simulink model "ARC_DTm"  (R2025b)
settings: Solver=FixedStepAuto  StartTime=0.0  StopTime=10080  FixedStep=1  RelTol=1e-3
PreLoadFcn:
  | %For Preload, set the working path
  | modelFolder = fileparts(which(bdroot));
  | addpath(genpath(modelFolder));
StartFcn:
  | tic
StopFcn:
  | fprintf("Sim Time: %.02f min", toc/60)
values from neighbouring files (symbols this model uses):
  batteryScenario = p.batteryScenario    [RUNSIM_ParameterSweep.m]    (also in _RUNSIM_ParameterSweep.m)
  Electricity_SalePriceModifier = 50/100    (= 0.5)    [RUNSIM_ParameterSweep.m]    (also in _RUNSIM_ParameterSweep.m)
  LUT = LUT_load.gamLUT    [RUNSIM_ParameterSweep.m]    (also in _RUNSIM_ParameterSweep.m)
  minimum_UF_system_flow = 5833    [RUNSIM_ParameterSweep.m]    (also in _RUNSIM_ParameterSweep.m)
  PROS1_recoveryrate = 61    [RUNSIM_ParameterSweep.m]    (also in _RUNSIM_ParameterSweep.m)
  PROS2_recoveryrate = 62    [RUNSIM_ParameterSweep.m]    (also in _RUNSIM_ParameterSweep.m)
  ROstabilization_time = p.ROstabilization_time    [RUNSIM_ParameterSweep.m]    (also in _RUNSIM_ParameterSweep.m)
  solarModifier = maximum_solar_generation / 300    [RUNSIM_ParameterSweep.m]    (also in _RUNSIM_ParameterSweep.m)
  TSRO_recoveryrate = 51    [RUNSIM_ParameterSweep.m]    (also in _RUNSIM_ParameterSweep.m)
  UF_RecoveryRate = 96    [RUNSIM_ParameterSweep.m]    (also in _RUNSIM_ParameterSweep.m)
undefined symbols (not defined in the file or in its folder): A_PROS1, A_PROS2, A_TSRO, B_PROS1, B_PROS2, B_TSRO, BW_Max_Time, BW_Max_Vol_gal, CEB_Max_Time, CEB_Max_Vol_gal, CIP_Max_Time, E, FF, h, L, w
libraries: simulink x40
(part 2 of 11)

== system ARC_DTm/PROS2_1 ==
  note: Units needed:
      | u = cm/sec
      | dh = cm
      | Concentrations = g/L
      | Jw_prev = L/m2/min
      |  = Q (Lpm) / Atot(m2)
      | T = oC
      | q = cm/sec =
      | Q (m3/sec) / Atot (m2)
  Inflow : Inport
  Brine Flow (gpm) : Sum  Inputs=-+
  Bus Creator : BusCreator  Inputs=2
  Bus Creator1 : BusCreator  Inputs=3
  Bus Selector : BusSelector  OutputSignals=S2 Feed Pressure (bar),Feed Temperature (oC),PROS1_1_BrineConductivity_gL,PROS1_1_BrineFlow_gpm
  Bus Selector1 : BusSelector  OutputSignals=PROS2_A,PROS2_B,PROS2_Area_m2
  Channel Area (m2) : Product  Inputs=4
  Check Valve1 : Saturate  UpperLimit=Inf  LowerLimit=0
  Check Valve2 : Saturate  UpperLimit=Inf  LowerLimit=0
  Elements per Vessel : Constant  Value=7
  Feed Channel Height (m) : Constant  Value=L
  Fouling Factor : Constant  Value=1-FF
  Gain : Gain  Gain=3.785
  Initial units : Gain  Gain=10^-8
  Jw_Previous : Memory  InitialCondition=.2949
  "L -> gal" : Gain  Gain=1/3.785
  L>m3 : Gain  Gain=1/1000
  MATLAB Function1 : MATLAB Function  TreatAsAtomicUnit=on
  MATLAB Function2 : MATLAB Function  TreatAsAtomicUnit=on
  Membrane Width (m) : Constant  Value=w
  Min : MinMax  Inputs=2
  Minus : Sum  Inputs=+-|
  Number of Vessels : Constant  Value=40
  Pa > Bar : Gain  Gain=100000
  Permeate Flow (gpm) : Product
  Product : Product  Inputs=*/
  Product2 : Product
  Q (L/min) : Gain  Gain=3.785
  Scope : Scope
      settings: ActiveDisplayYMinimum=-1  ActiveDisplayYMaximum=1  DataLoggingVariableName=ScopeData76
  Scope5 : Scope  NumInputPorts=3
      settings: ActiveDisplayYMinimum=-21.471979594450474  ActiveDisplayYMaximum=418.08306953365  DataLoggingVariableName=ScopeData74
  Spacer Thickness (mm) : Constant  Value=h
  Subsystem : Subsystem
  bar>psi : Gain  Gain=1/.069
  cperm_previous : Memory  InitialCondition=.008
  gpm > L : Gain  Gain=3.785
  initial Units : Gain  Gain=10^-11
  m/min > cm/sec : Gain  Gain=100/60
  m3 > L : Gain  Gain=1000
  m3 > L1 : Gain  Gain=1000
  m>cm : Gain  Gain=100
  m>mm : Gain  Gain=1000
  mm>  cm : Gain  Gain=.1
  mm>m : Gain  Gain=.001
  psi to Bar : Gain  Gain=.069
  s > min : Gain  Gain=60
  s > min1 : Gain  Gain=60
  PROS2_Permeate : Outport
  PROS2_Brine : Outport  Port=2
  tag scope: PROS2_1_deltaPi=global
  wires:
  m/min > cm/sec/1 -> Subsystem/11(u)
  [PROS2_MembraneConstants] -> Bus Selector1/1
  m3 > L1/1 -> s > min1/1
  Bus Selector/1 -> bar>psi/1, Subsystem/2(<S2 Feed Pressure (bar)>), Scope/1, Min/1  "<S2 Feed Pressure (bar)>"
  Bus Selector1/3 -> Permeate Flow (gpm)/2  "<PROS2_Area_m2>"
  Membrane Width (m)/1 -> Channel Area (m2)/1, m>mm/1
  [RO_PermeatePressure] -> psi to Bar/1  "Permeate Pressure (psi)"
  Inflow/1 -> Bus Selector/1
  Bus Selector1/1 -> initial Units/1  "<PROS2_A>"
  Bus Selector1/2 -> Initial units/1  "<PROS2_B>"
  Permeate Flow (gpm)/1 -> Check Valve2/1  "PROS2_1_PermeateFlow_gpm"
  Bus Selector/2 -> Subsystem/1(<Feed Temperature (oC)>)  "<Feed Temperature (oC)>"
  Bus Selector/3 -> MATLAB Function2/5(cfeed), Subsystem/6(<S2 Feed Salinity (g/L)>)  "<PROS1_1_BrineConductivity_gL>"
  Bus Selector/4 -> Q (L/min)/1, Brine Flow (gpm)/2  "<PROS1_1_BrineFlow_gpm>"
  Product/1 -> m/min > cm/sec/1
  psi to Bar/1 -> Min/2  "Pressure (bar)"
  MATLAB Function2/1(cbrine) -> Bus Creator1/2, Scope5/2  "PROS2_1_BrineConductivity_gL"
  initial Units/1 -> m3 > L/1
  Initial units/1 -> m3 > L1/1
  Spacer Thickness (mm)/1 -> MATLAB Function1/2(h), mm>m/1
  m3 > L/1 -> s > min/1
  Min/1 -> Subsystem/3(Pperm)
  mm>m/1 -> Channel Area (m2)/2
  Channel Area (m2)/1 -> Product/2
  Q (L/min)/1 -> MATLAB Function2/4(Qfeed), L>m3/1  "Qtot (L/min)"
  Bus Creator/1 -> PROS2_Permeate/1  "PRO1_PermeateFlow"
  Number of Vessels/1 -> Channel Area (m2)/3
  s > min/1 -> Pa > Bar/1
  Elements per Vessel/1 -> Channel Area (m2)/4
  s > min1/1 -> Subsystem/5(Salt Perm (L/m2/min))  "Salt Perm (L/m2/min)"
  Fouling Factor/1 -> Product2/2
  m>mm/1 -> MATLAB Function1/1(W)
  L>m3/1 -> Product/1
  Pa > Bar/1 -> Product2/1  "Water Perm (L/m2/min/Bar)"
  MATLAB Function1/1(dh) -> mm>  cm/1
  Feed Channel Height (m)/1 -> m>cm/1
  Jw_Previous/1 -> Subsystem/8(Jw)  "Jw"
  cperm_previous/1 -> Subsystem/7(cperm)  "cperm"
  m>cm/1 -> Subsystem/10(L)
  Product2/1 -> Subsystem/4(Water Perm (L/m2/min/Bar))  "Water Perm (L/m2/min/Bar)"
  Gain/1 -> MATLAB Function2/2(Qperm)  "Predicted Permeate Flow (L/min)"
  mm>  cm/1 -> Subsystem/9(dh)
  Bus Creator1/1 -> PROS2_Brine/1  "PROS2_Feedwater"
  bar>psi/1 -> Minus/1  "PROS2_1_ConcentratePressure_psi"
  Subsystem/1(Permeate Flux Rate (L/min/m2)) -> Jw_Previous/1, "L -> gal"/1  "Permeate Flux Rate* (L/min.m2)"
  Subsystem/2(Permeate Salinity g/L) -> Bus Creator/2, MATLAB Function2/1(cperm), cperm_previous/1  "PROS2_1_PermeateSalinity_gL"
  "L -> gal"/1 -> Permeate Flow (gpm)/1
  Subsystem/3(deltaPi_bar) -> [PROS2_1_deltaPi]
  Brine Flow (gpm)/1 -> Check Valve1/1  "PROS2_1_BrineFlow_gpm"
  gpm > L/1 -> MATLAB Function2/3(Qbrine)
  [PROS2_Suction_PressureDrop_psi] -> Minus/2
  Minus/1 -> Scope5/3, Bus Creator1/3  "PROS2_1_ConcentratePressure_psi"
  Check Valve1/1 -> Bus Creator1/1, Scope5/1, gpm > L/1  "PROS2_1_BrineFlow_gpm"
  Check Valve2/1 -> Bus Creator/1, Gain/1, Brine Flow (gpm)/1  "PROS2_1_PermeateFlow_gpm"

== system ARC_DTm/PROS2_1_Pump ==
  note: Determine Needed Added Pressure
  note: gpm / (gpm/psi*ft2) / ft2
  S2 Feed Flow Rate (gpm) : Inport
  Bar > psi : Gain  Gain=1/.069
  Bus Creator : BusCreator  Inputs=4
  Bus Selector : BusSelector  OutputSignals=PROS2_A,PROS2_Area_m2
  Bus Selector1 : BusSelector  OutputSignals=PROS1_1_BrineFlow_gpm,PROS1_1_BrineConductivity_gL,PROS1_1_ConcentratePressure_psi
  Constant2 : Constant  Value=0
  Constant4 : Constant  Value=0
  Gain : Gain  Gain=.01
  Gain3 : Gain  Gain=10.76
  MATLAB Function1 : MATLAB Function  TreatAsAtomicUnit=on
  Max : MinMax  Function=max  Inputs=2
  Memory : Memory  InitialCondition=15
  PROS2_1_recoveryrate_per : Constant  Value=62
  Pa > psi : Gain  Gain=6895
  Product : Product  Inputs=**/
  Product1 : Product
  Sum : Sum  Inputs=|-+
  Sum1 : Sum  Inputs=|++
  Sum2 : Sum  Inputs=|++
  Sum3 : Sum  Inputs=|+-
  Switch : Switch  Criteria=u2 > Threshold  Threshold=1  SaturateOnIntegerOverflow=off  InputSameDT=off
  Switch1 : Switch  Criteria=u2 > Threshold  Threshold=1  SaturateOnIntegerOverflow=off  InputSameDT=off
  m2 > ft2 : Gain  Gain=1/10.76
  m3 > gal : Gain  Gain=264.2
  m3/m2/s/Pa : Gain  Gain=10^-11
  psi to Bar : Gain  Gain=.069
  psi>ft : Gain  Gain=2.31
  s > min : Gain  Gain=60
  PROS2_1_Feedwater : Outport
  tag scope: PROS2_1_Power_kW=global
  wires:
  S2 Feed Flow Rate (gpm)/1 -> Bus Selector1/1  "InflowRate (gpm)"
  Sum1/1 -> Sum2/1  "Net Opposing Pressure (psi)"
  [PROS2_MembraneConstants] -> Bus Selector/1
  Pa > psi/1 -> m2 > ft2/1  "Water Perm (gpm/m2/bar)"
  Sum2/1 -> psi to Bar/1, Sum/2  "PROS2_1_FeedPressure_psi"
  m3 > gal/1 -> s > min/1
  [T] -> Bus Creator/2  "Feed Temperature (oC)"
  Memory/1 -> Sum1/1
  Product/1 -> Sum2/2  "PROS2_1_RequiredNDP_psi"
  PROS2_1_recoveryrate_per/1 -> Gain/1
  psi to Bar/1 -> Bus Creator/4  "S2 Feed Pressure (bar)"
  Gain3/1 -> Product1/2  "PROS2_Area_ft2"
  m2 > ft2/1 -> Product1/1  "PROS2_WaterPermeability_gpm_psi_ft2"
  Sum/1 -> psi>ft/1
  m3/m2/s/Pa/1 -> m3 > gal/1
  Bus Selector/1 -> m3/m2/s/Pa/1  "<PROS2_A>"
  Product1/1 -> Product/3
  [PROS2_1_deltaPi] -> Bar > psi/1
  Gain/1 -> Product/2
  s > min/1 -> Pa > psi/1
  Bar > psi/1 -> Memory/1
  Bus Creator/1 -> PROS2_1_Feedwater/1
  psi>ft/1 -> MATLAB Function1/2(h_des)
  Bus Selector1/2 -> Bus Creator/1  "<PROS1_1_BrineConductivity_gL>"
  Max/1 -> Sum3/1
  Bus Selector/2 -> Gain3/1  "<PROS2_Area_m2>"
  Sum3/1 -> Sum/1
  [PROS2_Suction_PressureDrop_psi] -> Switch1/1
  MATLAB Function1/2(power) -> [PROS2_1_Power_kW]  "PROS2_1_Power_kW"
  Bus Selector1/3 -> Max/1  "<PROS1_1_ConcentratePressure_psi>"
  Constant2/1 -> Switch1/3, Max/2
  Bus Selector1/1 -> Switch1/2, MATLAB Function1/1(Q_des), Bus Creator/3, Switch/2, Product/1  "<PROS1_1_BrineFlow_gpm>"
  [RO_PermeatePressure] -> Switch/1
  Constant4/1 -> Switch/3
  Switch/1 -> Sum1/2
  Switch1/1 -> Sum3/2

== system ARC_DTm/PROS2_2 ==
  note: Units needed:
      | u = cm/sec
      | dh = cm
      | Concentrations = g/L
      | Jw_prev = L/m2/min
      |  = Q (Lpm) / Atot(m2)
      | T = oC
      | q = cm/sec =
      | Q (m3/sec) / Atot (m2)
  Inflow : Inport
  Brine Flow (gpm) : Sum  Inputs=-+
  Bus Creator : BusCreator  Inputs=2
  Bus Creator1 : BusCreator  Inputs=3
  Bus Selector : BusSelector  OutputSignals=S2 Feed Pressure (bar),Feed Temperature (oC),PROS1_2_BrineConductivity_gL,PROS1_2_BrineFlow_gpm
  Bus Selector1 : BusSelector  OutputSignals=PROS2_A,PROS2_B,PROS2_Area_m2
  Channel Area (m2) : Product  Inputs=4
  Check Valve : Saturate  UpperLimit=Inf  LowerLimit=0
  Check Valve1 : Saturate  UpperLimit=Inf  LowerLimit=0
  Elements per Vessel : Constant  Value=7
  Feed Channel Height (m) : Constant  Value=L
  Fouling Factor : Constant  Value=1-FF
  Gain : Gain  Gain=3.785
  Initial units : Gain  Gain=10^-8
  Jw_Previous : Memory  InitialCondition=.2949
  "L -> gal" : Gain  Gain=1/3.785
  L>m3 : Gain  Gain=1/1000
  MATLAB Function1 : MATLAB Function  TreatAsAtomicUnit=on
  MATLAB Function2 : MATLAB Function  TreatAsAtomicUnit=on
  Membrane Width (m) : Constant  Value=w
  Min : MinMax  Inputs=2
  Minus : Sum  Inputs=+-|
  Number of Vessels : Constant  Value=40
  Pa > Bar : Gain  Gain=100000
  Permeate Flow (gpm) : Product
  Product : Product  Inputs=*/
  Product2 : Product
  Q (L/min) : Gain  Gain=3.785
  Scope : Scope
      settings: ActiveDisplayYMinimum=-1  ActiveDisplayYMaximum=1  DataLoggingVariableName=ScopeData76
  Scope5 : Scope  NumInputPorts=3
      settings: ActiveDisplayYMinimum=-102.45583996757739  ActiveDisplayYMaximum=443.57810434622803  DataLoggingVariableName=ScopeData74
  Spacer Thickness (mm) : Constant  Value=h
  Subsystem : Subsystem
  bar>psi : Gain  Gain=1/.069
  cperm_previous : Memory  InitialCondition=.008
  gpm > L : Gain  Gain=3.785
  initial Units : Gain  Gain=10^-11
  m/min > cm/sec : Gain  Gain=100/60
  m3 > L : Gain  Gain=1000
  m3 > L1 : Gain  Gain=1000
  m>cm : Gain  Gain=100
  m>mm : Gain  Gain=1000
  mm>  cm : Gain  Gain=.1
  mm>m : Gain  Gain=.001
  psi to Bar : Gain  Gain=.069
  s > min : Gain  Gain=60
  s > min1 : Gain  Gain=60
  PROS2_Permeate : Outport
  PROS2_Brine : Outport  Port=2
  tag scope: PROS2_2_deltaPi=global
  wires:
  m/min > cm/sec/1 -> Subsystem/11(u)
  [PROS2_MembraneConstants] -> Bus Selector1/1
  m3 > L1/1 -> s > min1/1
  Bus Selector/1 -> bar>psi/1, Subsystem/2(<S2 Feed Pressure (bar)>), Scope/1, Min/1  "<S2 Feed Pressure (bar)>"
  Bus Selector1/3 -> Permeate Flow (gpm)/2  "<PROS2_Area_m2>"
  Membrane Width (m)/1 -> Channel Area (m2)/1, m>mm/1
  [RO_PermeatePressure] -> psi to Bar/1  "Permeate Pressure (psi)"
  Inflow/1 -> Bus Selector/1
  Bus Selector1/1 -> initial Units/1  "<PROS2_A>"
  Bus Selector1/2 -> Initial units/1  "<PROS2_B>"
  Permeate Flow (gpm)/1 -> Check Valve/1  "PROS2_2_PermeateFlow_gpm"
  Bus Selector/2 -> Subsystem/1(<Feed Temperature (oC)>)  "<Feed Temperature (oC)>"
  Bus Selector/3 -> MATLAB Function2/5(cfeed), Subsystem/6(<S2 Feed Salinity (g/L)>)  "<PROS1_2_BrineConductivity_gL>"
  Bus Selector/4 -> Q (L/min)/1, Brine Flow (gpm)/2  "<PROS1_2_BrineFlow_gpm>"
  Product/1 -> m/min > cm/sec/1
  psi to Bar/1 -> Min/2  "Pressure (bar)"
  MATLAB Function2/1(cbrine) -> Bus Creator1/2, Scope5/2  "PROS2_2_BrineConductivity_gL"
  initial Units/1 -> m3 > L/1
  Initial units/1 -> m3 > L1/1
  Spacer Thickness (mm)/1 -> MATLAB Function1/2(h), mm>m/1
  m3 > L/1 -> s > min/1
  Min/1 -> Subsystem/3(Pperm)
  mm>m/1 -> Channel Area (m2)/2
  Channel Area (m2)/1 -> Product/2
  Q (L/min)/1 -> MATLAB Function2/4(Qfeed), L>m3/1  "Qtot (L/min)"
  Bus Creator/1 -> PROS2_Permeate/1  "PRO1_PermeateFlow"
  Number of Vessels/1 -> Channel Area (m2)/3
  s > min/1 -> Pa > Bar/1
  Elements per Vessel/1 -> Channel Area (m2)/4
  s > min1/1 -> Subsystem/5(Salt Perm (L/m2/min))  "Salt Perm (L/m2/min)"
  Fouling Factor/1 -> Product2/2
  m>mm/1 -> MATLAB Function1/1(W)
  L>m3/1 -> Product/1
  Pa > Bar/1 -> Product2/1  "Water Perm (L/m2/min/Bar)"
  MATLAB Function1/1(dh) -> mm>  cm/1
  Feed Channel Height (m)/1 -> m>cm/1
  Jw_Previous/1 -> Subsystem/8(Jw)  "Jw"
  cperm_previous/1 -> Subsystem/7(cperm)  "cperm"
  m>cm/1 -> Subsystem/10(L)
  Product2/1 -> Subsystem/4(Water Perm (L/m2/min/Bar))  "Water Perm (L/m2/min/Bar)"
  Gain/1 -> MATLAB Function2/2(Qperm)  "Predicted Permeate Flow (L/min)"
  mm>  cm/1 -> Subsystem/9(dh)
  Bus Creator1/1 -> PROS2_Brine/1  "PROS2_Feedwater"
  bar>psi/1 -> Minus/1  "PROS2_2_ConcentratePressure_psi"
  Subsystem/1(Permeate Flux Rate (L/min/m2)) -> Jw_Previous/1, "L -> gal"/1  "Permeate Flux Rate* (L/min.m2)"
  Subsystem/2(Permeate Salinity g/L) -> Bus Creator/2, MATLAB Function2/1(cperm), cperm_previous/1  "PROS2_2_PermeateSalinity_gL"
  "L -> gal"/1 -> Permeate Flow (gpm)/1
  Subsystem/3(deltaPi_bar) -> [PROS2_2_deltaPi]
  Brine Flow (gpm)/1 -> Check Valve1/1  "PROS2_2_BrineFlow_gpm"
  gpm > L/1 -> MATLAB Function2/3(Qbrine)
  [PROS2_Suction_PressureDrop_psi] -> Minus/2
  Minus/1 -> Scope5/3, Bus Creator1/3  "PROS2_2_ConcentratePressure_psi"
  Check Valve/1 -> Bus Creator/1, Gain/1, Brine Flow (gpm)/1  "PROS2_2_PermeateFlow_gpm"
  Check Valve1/1 -> Bus Creator1/1, Scope5/1, gpm > L/1  "PROS2_2_BrineFlow_gpm"

== system ARC_DTm/PROS2_2_Pump ==
  note: Determine Needed Added Pressure
  note: gpm / (gpm/psi*ft2) / ft2
  S2 Feed Flow Rate (gpm) : Inport
  Bar > psi : Gain  Gain=1/.069
  Bus Creator : BusCreator  Inputs=4
  Bus Selector : BusSelector  OutputSignals=PROS2_A,PROS2_Area_m2
  Bus Selector1 : BusSelector  OutputSignals=PROS1_2_BrineFlow_gpm,PROS1_2_BrineConductivity_gL,PROS1_2_ConcentratePressure_psi
  Constant2 : Constant  Value=0
  Constant4 : Constant  Value=0
  Gain : Gain  Gain=.01
  Gain3 : Gain  Gain=10.76
  MATLAB Function1 : MATLAB Function  TreatAsAtomicUnit=on
  Max : MinMax  Function=max  Inputs=2
  Memory : Memory  InitialCondition=15
  PROS2_2_recoveryrate_per : Constant  Value=62
  Pa > psi : Gain  Gain=6895
  Product : Product  Inputs=**/
  Product1 : Product
  Sum : Sum  Inputs=|-+
  Sum1 : Sum  Inputs=|++
  Sum2 : Sum  Inputs=|++
  Sum3 : Sum  Inputs=|+-
  Switch : Switch  Criteria=u2 > Threshold  Threshold=1  SaturateOnIntegerOverflow=off  InputSameDT=off
  Switch1 : Switch  Criteria=u2 > Threshold  Threshold=1  SaturateOnIntegerOverflow=off  InputSameDT=off
  m2 > ft2 : Gain  Gain=1/10.76
  m3 > gal : Gain  Gain=264.2
  m3/m2/s/Pa : Gain  Gain=10^-11
  psi to Bar : Gain  Gain=.069
  psi>ft : Gain  Gain=2.31
  s > min : Gain  Gain=60
  PROS2_2_Feedwater : Outport
  tag scope: PROS2_2_Power_kW=global
  wires:
  S2 Feed Flow Rate (gpm)/1 -> Bus Selector1/1  "InflowRate (gpm)"
  Sum1/1 -> Sum2/1  "Net Opposing Pressure (psi)"
  [PROS2_MembraneConstants] -> Bus Selector/1
  Pa > psi/1 -> m2 > ft2/1  "Water Perm (gpm/m2/bar)"
  Sum2/1 -> psi to Bar/1, Sum/2  "PROS2_2_FeedPressure_psi"
  m3 > gal/1 -> s > min/1
  [T] -> Bus Creator/2  "Feed Temperature (oC)"
  Memory/1 -> Sum1/1
  Product/1 -> Sum2/2  "PROS2_2_RequiredNDP_psi"
  PROS2_2_recoveryrate_per/1 -> Gain/1
  psi to Bar/1 -> Bus Creator/4  "S2 Feed Pressure (bar)"
  Gain3/1 -> Product1/2  "PROS2_Area_ft2"
  m2 > ft2/1 -> Product1/1  "PROS2_WaterPermeability_gpm_psi_ft2"
  Sum/1 -> psi>ft/1
  m3/m2/s/Pa/1 -> m3 > gal/1
  Bus Selector/1 -> m3/m2/s/Pa/1  "<PROS2_A>"
  Product1/1 -> Product/3
  [PROS2_2_deltaPi] -> Bar > psi/1
  Gain/1 -> Product/2
  s > min/1 -> Pa > psi/1
  Bar > psi/1 -> Memory/1
  Bus Creator/1 -> PROS2_2_Feedwater/1
  psi>ft/1 -> MATLAB Function1/2(h_des)
  Bus Selector1/2 -> Bus Creator/1  "<PROS1_2_BrineConductivity_gL>"
  Max/1 -> Sum3/1
  Bus Selector/2 -> Gain3/1  "<PROS2_Area_m2>"
  Sum3/1 -> Sum/1
  [PROS2_Suction_PressureDrop_psi] -> Switch1/1
  MATLAB Function1/2(power) -> [PROS2_2_Power_kW]  "PROS2_2_Power_kW"
  Bus Selector1/3 -> Max/1  "<PROS1_2_ConcentratePressure_psi>"
  Constant2/1 -> Switch1/3, Max/2
  Bus Selector1/1 -> Switch1/2, MATLAB Function1/1(Q_des), Bus Creator/3, Switch/2, Product/1  "<PROS1_2_BrineFlow_gpm>"
  [RO_PermeatePressure] -> Switch/1
  Constant4/1 -> Switch/3
  Switch/1 -> Sum1/2
  Switch1/1 -> Sum3/2

== system ARC_DTm/PROS2_3 ==
  note: Units needed:
      | u = cm/sec
      | dh = cm
      | Concentrations = g/L
      | Jw_prev = L/m2/min
      |  = Q (Lpm) / Atot(m2)
      | T = oC
      | q = cm/sec =
      | Q (m3/sec) / Atot (m2)
  Inflow : Inport
  Brine Flow (gpm) : Sum  Inputs=-+
  Bus Creator : BusCreator  Inputs=2
  Bus Creator1 : BusCreator  Inputs=3
  Bus Selector : BusSelector  OutputSignals=S2 Feed Pressure (bar),Feed Temperature (oC),PROS1_3_BrineConductivity_gL,PROS1_3_BrineFlow_gpm
  Bus Selector1 : BusSelector  OutputSignals=PROS2_A,PROS2_B,PROS2_Area_m2
  Channel Area (m2) : Product  Inputs=4
  Check Valve : Saturate  UpperLimit=Inf  LowerLimit=0
  Check Valve1 : Saturate  UpperLimit=Inf  LowerLimit=0
  Elements per Vessel : Constant  Value=7
  Feed Channel Height (m) : Constant  Value=L
  Fouling Factor : Constant  Value=1-FF
  Gain : Gain  Gain=3.785
  Initial units : Gain  Gain=10^-8
  Jw_Previous : Memory  InitialCondition=.2949
  "L -> gal" : Gain  Gain=1/3.785
  L>m3 : Gain  Gain=1/1000
  MATLAB Function1 : MATLAB Function  TreatAsAtomicUnit=on
  MATLAB Function2 : MATLAB Function  TreatAsAtomicUnit=on
  Membrane Width (m) : Constant  Value=w
  Min : MinMax  Inputs=2
  Minus : Sum  Inputs=+-|
  Number of Vessels : Constant  Value=40
  Pa > Bar : Gain  Gain=100000
  Permeate Flow (gpm) : Product
  Product : Product  Inputs=*/
  Product2 : Product
  Q (L/min) : Gain  Gain=3.785
  Scope : Scope
      settings: ActiveDisplayYMinimum=-1  ActiveDisplayYMaximum=1  DataLoggingVariableName=ScopeData76
  Spacer Thickness (mm) : Constant  Value=h
  Subsystem : Subsystem
  bar>psi : Gain  Gain=1/.069
  cperm_previous : Memory  InitialCondition=.008
  gpm > L : Gain  Gain=3.785
  initial Units : Gain  Gain=10^-11
  m/min > cm/sec : Gain  Gain=100/60
  m3 > L : Gain  Gain=1000
  m3 > L1 : Gain  Gain=1000
  m>cm : Gain  Gain=100
  m>mm : Gain  Gain=1000
  mm>  cm : Gain  Gain=.1
  mm>m : Gain  Gain=.001
  psi to Bar : Gain  Gain=.069
  s > min : Gain  Gain=60
  s > min1 : Gain  Gain=60
  PROS2_Permeate : Outport
  PROS2_Brine : Outport  Port=2
  tag scope: PROS2_3_deltaPi=global
  wires:
  m/min > cm/sec/1 -> Subsystem/11(u)
  [PROS2_MembraneConstants] -> Bus Selector1/1
  m3 > L1/1 -> s > min1/1
  Bus Selector/1 -> bar>psi/1, Subsystem/2(<S2 Feed Pressure (bar)>), Scope/1, Min/1  "<S2 Feed Pressure (bar)>"
  Bus Selector1/3 -> Permeate Flow (gpm)/2  "<PROS2_Area_m2>"
  Membrane Width (m)/1 -> Channel Area (m2)/1, m>mm/1
  [RO_PermeatePressure] -> psi to Bar/1  "Permeate Pressure (psi)"
  Inflow/1 -> Bus Selector/1
  Bus Selector1/1 -> initial Units/1  "<PROS2_A>"
  Bus Selector1/2 -> Initial units/1  "<PROS2_B>"
  Permeate Flow (gpm)/1 -> Check Valve1/1  "PROS2_3_PermeateFlow_gpm"
  Bus Selector/2 -> Subsystem/1(<Feed Temperature (oC)>)  "<Feed Temperature (oC)>"
  Bus Selector/3 -> MATLAB Function2/5(cfeed), Subsystem/6(<S2 Feed Salinity (g/L)>)  "<PROS1_3_BrineConductivity_gL>"
  Bus Selector/4 -> Q (L/min)/1, Brine Flow (gpm)/2  "<PROS1_3_BrineFlow_gpm>"
  Product/1 -> m/min > cm/sec/1
  psi to Bar/1 -> Min/2  "Pressure (bar)"
  MATLAB Function2/1(cbrine) -> Bus Creator1/2  "PROS2_3_BrineConductivity_gL"
  initial Units/1 -> m3 > L/1
  Initial units/1 -> m3 > L1/1
  Spacer Thickness (mm)/1 -> MATLAB Function1/2(h), mm>m/1
  m3 > L/1 -> s > min/1
  Min/1 -> Subsystem/3(Pperm)
  mm>m/1 -> Channel Area (m2)/2
  Channel Area (m2)/1 -> Product/2
  Q (L/min)/1 -> MATLAB Function2/4(Qfeed), L>m3/1  "Qtot (L/min)"
  Bus Creator/1 -> PROS2_Permeate/1  "PRO1_PermeateFlow"
  Number of Vessels/1 -> Channel Area (m2)/3
  s > min/1 -> Pa > Bar/1
  Elements per Vessel/1 -> Channel Area (m2)/4
  s > min1/1 -> Subsystem/5(Salt Perm (L/m2/min))  "Salt Perm (L/m2/min)"
  Fouling Factor/1 -> Product2/2
  m>mm/1 -> MATLAB Function1/1(W)
  L>m3/1 -> Product/1
  Pa > Bar/1 -> Product2/1  "Water Perm (L/m2/min/Bar)"
  MATLAB Function1/1(dh) -> mm>  cm/1
  Feed Channel Height (m)/1 -> m>cm/1
  Jw_Previous/1 -> Subsystem/8(Jw)  "Jw"
  cperm_previous/1 -> Subsystem/7(cperm)  "cperm"
  m>cm/1 -> Subsystem/10(L)
  Product2/1 -> Subsystem/4(Water Perm (L/m2/min/Bar))  "Water Perm (L/m2/min/Bar)"
  Gain/1 -> MATLAB Function2/2(Qperm)  "Predicted Permeate Flow (L/min)"
  mm>  cm/1 -> Subsystem/9(dh)
  Bus Creator1/1 -> PROS2_Brine/1  "PROS2_Feedwater"
  bar>psi/1 -> Minus/1  "PROS2_3_ConcentratePressure_psi"
  Subsystem/1(Permeate Flux Rate (L/min/m2)) -> Jw_Previous/1, "L -> gal"/1  "Permeate Flux Rate* (L/min.m2)"
  Subsystem/2(Permeate Salinity g/L) -> Bus Creator/2, MATLAB Function2/1(cperm), cperm_previous/1  "PROS2_3_PermeateSalinity_gL"
  "L -> gal"/1 -> Permeate Flow (gpm)/1
  Subsystem/3(deltaPi_bar) -> [PROS2_3_deltaPi]
  Check Valve/1 -> Bus Creator1/1, gpm > L/1  "PROS2_3_BrineFlow_gpm"
  gpm > L/1 -> MATLAB Function2/3(Qbrine)
  [PROS2_Suction_PressureDrop_psi] -> Minus/2
  Minus/1 -> Bus Creator1/3  "PROS2_3_ConcentratePressure_psi"
  Brine Flow (gpm)/1 -> Check Valve/1  "PROS2_3_BrineFlow_gpm"
  Check Valve1/1 -> Bus Creator/1, Gain/1, Brine Flow (gpm)/1  "PROS2_3_PermeateFlow_gpm"

== system ARC_DTm/PROS2_3_Pump ==
  note: Determine Needed Added Pressure
  note: gpm / (gpm/psi*ft2) / ft2
  S2 Feed Flow Rate (gpm) : Inport
  Bar > psi : Gain  Gain=1/.069
  Bus Creator : BusCreator  Inputs=4
  Bus Selector : BusSelector  OutputSignals=PROS2_A,PROS2_Area_m2
  Bus Selector1 : BusSelector  OutputSignals=PROS1_3_BrineFlow_gpm,PROS1_3_BrineConductivity_gL,PROS1_3_ConcentratePressure_psi
  Constant2 : Constant  Value=0
  Constant4 : Constant  Value=0
  Gain : Gain  Gain=.01
  Gain3 : Gain  Gain=10.76
  MATLAB Function1 : MATLAB Function  TreatAsAtomicUnit=on
  Max : MinMax  Function=max  Inputs=2
  Memory : Memory  InitialCondition=15
  PROS2_3_recoveryrate_per : Constant  Value=62
  Pa > psi : Gain  Gain=6895
  Product : Product  Inputs=**/
  Product1 : Product
  Sum : Sum  Inputs=|-+
  Sum1 : Sum  Inputs=|++
  Sum2 : Sum  Inputs=|++
  Sum3 : Sum  Inputs=|+-
  Switch : Switch  Criteria=u2 > Threshold  Threshold=1  SaturateOnIntegerOverflow=off  InputSameDT=off
  Switch1 : Switch  Criteria=u2 > Threshold  Threshold=1  SaturateOnIntegerOverflow=off  InputSameDT=off
  m2 > ft2 : Gain  Gain=1/10.76
  m3 > gal : Gain  Gain=264.2
  m3/m2/s/Pa : Gain  Gain=10^-11
  psi to Bar : Gain  Gain=.069
  psi>ft : Gain  Gain=2.31
  s > min : Gain  Gain=60
  PROS2_3_Feedwater : Outport
  tag scope: PROS2_3_Power_kW=global
  wires:
  S2 Feed Flow Rate (gpm)/1 -> Bus Selector1/1  "InflowRate (gpm)"
  Sum1/1 -> Sum2/1  "Net Opposing Pressure (psi)"
  [PROS2_MembraneConstants] -> Bus Selector/1
  Pa > psi/1 -> m2 > ft2/1  "Water Perm (gpm/m2/bar)"
  Sum2/1 -> psi to Bar/1, Sum/2  "PROS2_3_FeedPressure_psi"
  m3 > gal/1 -> s > min/1
  [T] -> Bus Creator/2  "Feed Temperature (oC)"
  Memory/1 -> Sum1/1
  Product/1 -> Sum2/2  "PROS2_3_RequiredNDP_psi"
  PROS2_3_recoveryrate_per/1 -> Gain/1
  psi to Bar/1 -> Bus Creator/4  "S2 Feed Pressure (bar)"
  Gain3/1 -> Product1/2  "PROS2_Area_ft2"
  m2 > ft2/1 -> Product1/1  "PROS2_WaterPermeability_gpm_psi_ft2"
  Sum/1 -> psi>ft/1
  m3/m2/s/Pa/1 -> m3 > gal/1
  Bus Selector/1 -> m3/m2/s/Pa/1  "<PROS2_A>"
  Product1/1 -> Product/3
  [PROS2_3_deltaPi] -> Bar > psi/1
  Gain/1 -> Product/2
  s > min/1 -> Pa > psi/1
  Bar > psi/1 -> Memory/1
  Bus Creator/1 -> PROS2_3_Feedwater/1
  psi>ft/1 -> MATLAB Function1/2(h_des)
  Bus Selector1/2 -> Bus Creator/1  "<PROS1_3_BrineConductivity_gL>"
  Max/1 -> Sum3/1
  Bus Selector/2 -> Gain3/1  "<PROS2_Area_m2>"
  Sum3/1 -> Sum/1
  [PROS2_Suction_PressureDrop_psi] -> Switch1/1
  MATLAB Function1/2(power) -> [PROS2_3_Power_kW]  "PROS2_3_Power_kW"
  Bus Selector1/3 -> Max/1  "<PROS1_3_ConcentratePressure_psi>"
  Constant2/1 -> Switch1/3, Max/2
  Bus Selector1/1 -> Switch1/2, MATLAB Function1/1(Q_des), Bus Creator/3, Switch/2, Product/1  "<PROS1_3_BrineFlow_gpm>"
  [RO_PermeatePressure] -> Switch/1
  Constant4/1 -> Switch/3
  Switch/1 -> Sum1/2
  Switch1/1 -> Sum3/2

== system ARC_DTm/PROS2_4 ==
  note: Units needed:
      | u = cm/sec
      | dh = cm
      | Concentrations = g/L
      | Jw_prev = L/m2/min
      |  = Q (Lpm) / Atot(m2)
      | T = oC
      | q = cm/sec =
      | Q (m3/sec) / Atot (m2)
  Inflow : Inport
  Brine Flow (gpm) : Sum  Inputs=-+
  Bus Creator : BusCreator  Inputs=2
  Bus Creator1 : BusCreator  Inputs=3
  Bus Selector : BusSelector  OutputSignals=S2 Feed Pressure (bar),Feed Temperature (oC),PROS1_4_BrineConductivity_gL,PROS1_4_BrineFlow_gpm
  Bus Selector1 : BusSelector  OutputSignals=PROS2_A,PROS2_B,PROS2_Area_m2
  Channel Area (m2) : Product  Inputs=4
  Check Valve : Saturate  UpperLimit=Inf  LowerLimit=0
  Check Valve2 : Saturate  UpperLimit=Inf  LowerLimit=0
  Elements per Vessel : Constant  Value=7
  Feed Channel Height (m) : Constant  Value=L
  Fouling Factor : Constant  Value=1-FF
  Gain : Gain  Gain=3.785
  Initial units : Gain  Gain=10^-8
  Jw_Previous : Memory  InitialCondition=.2949
  "L -> gal" : Gain  Gain=1/3.785
  L>m3 : Gain  Gain=1/1000
  MATLAB Function1 : MATLAB Function  TreatAsAtomicUnit=on
  MATLAB Function2 : MATLAB Function  TreatAsAtomicUnit=on
  Membrane Width (m) : Constant  Value=w
  Min : MinMax  Inputs=2
  Minus : Sum  Inputs=+-|
  Number of Vessels : Constant  Value=40
  Pa > Bar : Gain  Gain=100000
  Permeate Flow (gpm) : Product
  Product : Product  Inputs=*/
  Product2 : Product
  Q (L/min) : Gain  Gain=3.785
  Scope : Scope
      settings: ActiveDisplayYMinimum=-1  ActiveDisplayYMaximum=1  DataLoggingVariableName=ScopeData76
  Scope1 : Scope  NumInputPorts=2
      settings: ActiveDisplayYMinimum=-394.68314201102044  ActiveDisplayYMaximum=456.3600674223589  DataLoggingVariableName=ScopeData35
  Spacer Thickness (mm) : Constant  Value=h
  Subsystem : Subsystem
  bar>psi : Gain  Gain=1/.069
  cperm_previous : Memory  InitialCondition=.008
  gpm > L : Gain  Gain=3.785
  initial Units : Gain  Gain=10^-11
  m/min > cm/sec : Gain  Gain=100/60
  m3 > L : Gain  Gain=1000
  m3 > L1 : Gain  Gain=1000
  m>cm : Gain  Gain=100
  m>mm : Gain  Gain=1000
  mm>  cm : Gain  Gain=.1
  mm>m : Gain  Gain=.001
  psi to Bar : Gain  Gain=.069
  s > min : Gain  Gain=60
  s > min1 : Gain  Gain=60
  PROS2_Permeate : Outport
  PROS2_Brine : Outport  Port=2
  tag scope: PROS2_4_deltaPi=global
  wires:
  m/min > cm/sec/1 -> Subsystem/11(u)
  [PROS2_MembraneConstants] -> Bus Selector1/1
  m3 > L1/1 -> s > min1/1
  Bus Selector/1 -> bar>psi/1, Subsystem/2(<S2 Feed Pressure (bar)>), Scope/1, Min/1  "<S2 Feed Pressure (bar)>"
  Bus Selector1/3 -> Permeate Flow (gpm)/2  "<PROS2_Area_m2>"
  Membrane Width (m)/1 -> Channel Area (m2)/1, m>mm/1
  [RO_PermeatePressure] -> psi to Bar/1  "Permeate Pressure (psi)"
  Inflow/1 -> Bus Selector/1
  Bus Selector1/1 -> initial Units/1  "<PROS2_A>"
  Bus Selector1/2 -> Initial units/1  "<PROS2_B>"
  Permeate Flow (gpm)/1 -> Check Valve2/1  "PROS2_4_PermeateFlow_gpm"
  Bus Selector/2 -> Subsystem/1(<Feed Temperature (oC)>)  "<Feed Temperature (oC)>"
  Bus Selector/3 -> MATLAB Function2/5(cfeed), Subsystem/6(<S2 Feed Salinity (g/L)>)  "<PROS1_4_BrineConductivity_gL>"
  Bus Selector/4 -> Q (L/min)/1, Brine Flow (gpm)/2  "<PROS1_4_BrineFlow_gpm>"
  Product/1 -> m/min > cm/sec/1
  psi to Bar/1 -> Min/2  "Pressure (bar)"
  MATLAB Function2/1(cbrine) -> Scope1/2, Bus Creator1/2  "PROS2_4_BrineConductivity_gL"
  initial Units/1 -> m3 > L/1
  Initial units/1 -> m3 > L1/1
  Spacer Thickness (mm)/1 -> MATLAB Function1/2(h), mm>m/1
  m3 > L/1 -> s > min/1
  Min/1 -> Subsystem/3(Pperm)
  mm>m/1 -> Channel Area (m2)/2
  Channel Area (m2)/1 -> Product/2
  Q (L/min)/1 -> MATLAB Function2/4(Qfeed), L>m3/1  "Qtot (L/min)"
  Bus Creator/1 -> PROS2_Permeate/1  "PRO1_PermeateFlow"
  Number of Vessels/1 -> Channel Area (m2)/3
  s > min/1 -> Pa > Bar/1
  Elements per Vessel/1 -> Channel Area (m2)/4
  s > min1/1 -> Subsystem/5(Salt Perm (L/m2/min))  "Salt Perm (L/m2/min)"
  Fouling Factor/1 -> Product2/2
  m>mm/1 -> MATLAB Function1/1(W)
  L>m3/1 -> Product/1
  Pa > Bar/1 -> Product2/1  "Water Perm (L/m2/min/Bar)"
  MATLAB Function1/1(dh) -> mm>  cm/1
  Feed Channel Height (m)/1 -> m>cm/1
  Jw_Previous/1 -> Subsystem/8(Jw)  "Jw"
  cperm_previous/1 -> Subsystem/7(cperm)  "cperm"
  m>cm/1 -> Subsystem/10(L)
  Product2/1 -> Subsystem/4(Water Perm (L/m2/min/Bar))  "Water Perm (L/m2/min/Bar)"
  Gain/1 -> MATLAB Function2/2(Qperm)  "Predicted Permeate Flow (L/min)"
  mm>  cm/1 -> Subsystem/9(dh)
  Bus Creator1/1 -> PROS2_Brine/1  "PROS2_Feedwater"
  bar>psi/1 -> Minus/1  "PROS2_4_ConcentratePressure_psi"
  Subsystem/1(Permeate Flux Rate (L/min/m2)) -> Jw_Previous/1, "L -> gal"/1  "Permeate Flux Rate* (L/min.m2)"
  Subsystem/2(Permeate Salinity g/L) -> Bus Creator/2, MATLAB Function2/1(cperm), cperm_previous/1  "PROS2_4_PermeateSalinity_gL"
  "L -> gal"/1 -> Permeate Flow (gpm)/1
  Subsystem/3(deltaPi_bar) -> [PROS2_4_deltaPi]
  Check Valve/1 -> Bus Creator1/1, Scope1/1, gpm > L/1  "PROS2_4_BrineFlow_gpm"
  gpm > L/1 -> MATLAB Function2/3(Qbrine)
  [PROS2_Suction_PressureDrop_psi] -> Minus/2
  Minus/1 -> Bus Creator1/3  "PROS2_4_ConcentratePressure_psi"
  Brine Flow (gpm)/1 -> Check Valve/1  "PROS2_4_BrineFlow_gpm"
  Check Valve2/1 -> Brine Flow (gpm)/1, Bus Creator/1, Gain/1  "PROS2_4_PermeateFlow_gpm"

== system ARC_DTm/PROS2_4_Pump ==
  note: Determine Needed Added Pressure
  note: gpm / (gpm/psi*ft2) / ft2
  S2 Feed Flow Rate (gpm) : Inport
  Bar > psi : Gain  Gain=1/.069
  Bus Creator : BusCreator  Inputs=4
  Bus Selector : BusSelector  OutputSignals=PROS2_A,PROS2_Area_m2
  Bus Selector1 : BusSelector  OutputSignals=PROS1_4_BrineFlow_gpm,PROS1_4_BrineConductivity_gL,PROS1_4_ConcentratePressure_psi
  Constant2 : Constant  Value=0
  Constant4 : Constant  Value=0
  Gain : Gain  Gain=.01
  Gain3 : Gain  Gain=10.76
  MATLAB Function1 : MATLAB Function  TreatAsAtomicUnit=on
  Max : MinMax  Function=max  Inputs=2
  Memory : Memory  InitialCondition=15
  PROS2_4_recoveryrate_per : Constant  Value=62
  Pa > psi : Gain  Gain=6895
  Product : Product  Inputs=**/
  Product1 : Product
  Sum : Sum  Inputs=|-+
  Sum1 : Sum  Inputs=|++
  Sum2 : Sum  Inputs=|++
  Sum3 : Sum  Inputs=|+-
  Switch : Switch  Criteria=u2 > Threshold  Threshold=1  SaturateOnIntegerOverflow=off  InputSameDT=off
  Switch1 : Switch  Criteria=u2 > Threshold  Threshold=1  SaturateOnIntegerOverflow=off  InputSameDT=off
  m2 > ft2 : Gain  Gain=1/10.76
  m3 > gal : Gain  Gain=264.2
  m3/m2/s/Pa : Gain  Gain=10^-11
  psi to Bar : Gain  Gain=.069
  psi>ft : Gain  Gain=2.31
  s > min : Gain  Gain=60
  PROS2_4_Feedwater : Outport
  tag scope: PROS2_4_Power_kW=global
  wires:
  S2 Feed Flow Rate (gpm)/1 -> Bus Selector1/1  "InflowRate (gpm)"
  Sum1/1 -> Sum2/1  "Net Opposing Pressure (psi)"
  [PROS2_MembraneConstants] -> Bus Selector/1
  Pa > psi/1 -> m2 > ft2/1  "Water Perm (gpm/m2/bar)"
  Sum2/1 -> psi to Bar/1, Sum/2  "PROS2_4_FeedPressure_psi"
  m3 > gal/1 -> s > min/1
  [T] -> Bus Creator/2  "Feed Temperature (oC)"
  Memory/1 -> Sum1/1
  Product/1 -> Sum2/2  "PROS2_4_RequiredNDP_psi"
  PROS2_4_recoveryrate_per/1 -> Gain/1
  psi to Bar/1 -> Bus Creator/4  "S2 Feed Pressure (bar)"
  Gain3/1 -> Product1/2  "PROS2_Area_ft2"
  m2 > ft2/1 -> Product1/1  "PROS2_WaterPermeability_gpm_psi_ft2"
  Sum/1 -> psi>ft/1
  m3/m2/s/Pa/1 -> m3 > gal/1
  Bus Selector/1 -> m3/m2/s/Pa/1  "<PROS2_A>"
  Product1/1 -> Product/3
  [PROS2_4_deltaPi] -> Bar > psi/1
  Gain/1 -> Product/2
  s > min/1 -> Pa > psi/1
  Bar > psi/1 -> Memory/1
  Bus Creator/1 -> PROS2_4_Feedwater/1
  psi>ft/1 -> MATLAB Function1/2(h_des)
  Bus Selector1/2 -> Bus Creator/1  "<PROS1_4_BrineConductivity_gL>"
  Max/1 -> Sum3/1
  Bus Selector/2 -> Gain3/1  "<PROS2_Area_m2>"
  Sum3/1 -> Sum/1
  [PROS2_Suction_PressureDrop_psi] -> Switch1/1
  MATLAB Function1/2(power) -> [PROS2_4_Power_kW]  "PROS2_4_Power_kW"
  Bus Selector1/3 -> Max/1  "<PROS1_4_ConcentratePressure_psi>"
  Constant2/1 -> Switch1/3, Max/2
  Bus Selector1/1 -> Switch1/2, MATLAB Function1/1(Q_des), Bus Creator/3, Switch/2, Product/1  "<PROS1_4_BrineFlow_gpm>"
  [RO_PermeatePressure] -> Switch/1
  Constant4/1 -> Switch/3
  Switch/1 -> Sum1/2
  Switch1/1 -> Sum3/2

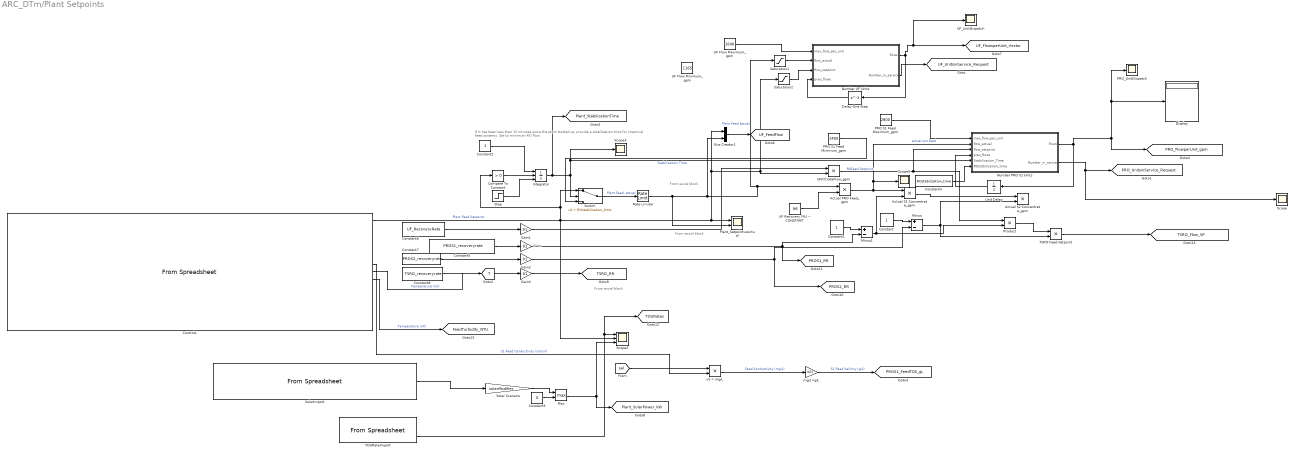
== system ARC_DTm/Plant Setpoints ==
  note: If it has been less than 15 minutes since the plant started up, provide a stabilization time for chemical feed systems.
      | Set to minimum RO flow.
  note: From excel block
  note: From excel block
  note: From excel block
  Actual PRO Feed_gpm : Product
  Actual S1 Concentrate_gpm : Product
  Actual S2 Concentrate_gpm : Product
  Bus Creator1 : BusCreator  Inputs=2
  Compare To Constant : simulink/Logic and Bit Operations/Compare To Constant  relop=>  const=0  OutDataTypeStr=boolean
  Constant : Constant
  Constant1 : Constant
  Constant2 : Constant
  Constant3 : Constant  Value=0
  Constant4 : Constant  Value=ROstabilization_time
  Constant5 : Constant  Value=PROS1_recoveryrate
  Constant6 : Constant  Value=UF_RecoveryRate
  Constant7 : Constant  Value=PROS2_recoveryrate
  Constant8 : Constant  Value=TSRO_recoveryrate
  Controls : FromSpreadsheet  FileName=OperationalScenarios.xlsx  SheetName=CompleteShutdown_TOU  SampleTime=1  InterpolationWithinTimeRange=Zero order hold
  Delay One Step : Delay  DelayLength=1
  Display : Display
  Gain{,1..3} (4 alike) : Gain  Gain=.01
  Integrator : Integrator  ExternalReset=rising  InitialConditionSource=external  InitialCondition=36
  Max : MinMax  Function=max  Inputs=2
  Minus : Sum  Inputs=+-
  Minus1 : Sum  Inputs=+-
  Number PRO S1 Units : MATLAB Function  TreatAsAtomicUnit=on
  Number UF Units : MATLAB Function  TreatAsAtomicUnit=on
  PRO S1 Feed Maximum_gpm : Constant  Value=2800
  PRO S1 Feed Minimum_gpm : Constant  Value=1400
  PRO_UnitDispatch : Scope
      settings: ActiveDisplayYMinimum=-164.53124999999994  ActiveDisplayYMaximum=2898.28125  DataLoggingVariableName=ScopeData57
  Plant_SetpointvsActual : Scope  NumInputPorts=2
      settings: TimeSpan=1440  Title=Plant Flow Setpoint vs. Actual  ActiveDisplayYMinimum=-1406.2499999999998  ActiveDisplayYMaximum=12656.25  DataLoggingVariableName=ScopeData8
  Product : Product
  Rate Limiter : RateLimiter  RisingSlewLimit=10056/85  FallingSlewLimit=-10056/37  SampleTimeMode=inherited  InitialCondition=8000
  Saturation1 : Saturate  UpperLimit=11000  LowerLimit=minimum_UF_system_flow
  Saturation2 : Saturate  UpperLimit=11000  LowerLimit=minimum_UF_system_flow
  Scope : Scope
      settings: ActiveDisplayYMinimum=-0.49999999999999989  ActiveDisplayYMaximum=4.5  DataLoggingVariableName=ScopeData12
  Scope2 : Scope  NumInputPorts=3
      settings: ActiveDisplayYMinimum=0.026983729999999997  ActiveDisplayYMaximum=0.04698373  DataLoggingVariableName=ScopeData10
  Scope3 : Scope
      settings: ActiveDisplayYMinimum=-281.74999999999989  ActiveDisplayYMaximum=3595.75  DataLoggingVariableName=ScopeData48
  Scope5 : Scope
      settings: ActiveDisplayYMinimum=4725  ActiveDisplayYMaximum=11475  DataLoggingVariableName=ScopeData58
  Solar Scenario : Gain  Gain=solarModifier
  SolarImport : FromSpreadsheet  FileName=C:\Users\joshl\Desktop\ARC_Complete\SolarSimulationData\SolarData_2021-06-10.xlsx  Range=D1:D1441  TreatFirstColumnAs=Data  SampleTime=1
  Step : Step  Before=ROstabilization_time+1  After=0  SampleTime=0
  Switch : Switch  Criteria=u2 > Threshold  Threshold=ROstabilization_time  SaturateOnIntegerOverflow=off  InputSameDT=off
  TOURateImport : FromSpreadsheet  FileName=_TOURates.xlsx  SheetName=ExistingTOU  TreatFirstColumnAs=Data  SampleTime=1
  TSRO Feed Setpoint : Product
  UF Flow Maximum_gpm : Constant  Value=1640
  UF Flow Minimum_gpm : Constant  Value=1165
  "UF Recovery (%) -- CONSTANT" : Constant  Value=.96
  UFFiltrateFlow_gpm : Product
  UF_UnitDispatch : Scope
      settings: ActiveDisplayYMinimum=-196.42857142857136  ActiveDisplayYMaximum=1767.8571428571427  DataLoggingVariableName=ScopeData67
  Unit Delay : UnitDelay  SampleTime=-1  HasFrameUpgradeWarning=on
  mg/L>g/L : Gain  Gain=.001
  uS > mg/L : Product
  tag scope: FeedTurbidity_NTU=global, PROS1_FeedTDS_gL=global, PROS1_RR=global, PROS2_RR=global, PRO_FlowperUnit_gpm=global, PRO_UnitsinService_Request=global, Plant_SolarPower_kW=global, Plant_StabilizationTime=global, T=global, TOURates=global, TSRO_Flow_SP=global, TSRO_RR=global, UF_FeedFlow=global, UF_FlowsperUnit_Vector=global, UF_UnitsinService_Request=global
  wires:
  "UF Recovery (%) -- CONSTANT"/1 -> Actual PRO Feed_gpm/2
  Actual PRO Feed_gpm/1 -> Scope5/1, Number PRO S1 Units/2(flow_actual), Actual S1 Concentrate_gpm/1  "actual pro feed"
  Constant5/1 -> Gain/1
  PRO S1 Feed Maximum_gpm/1 -> Number PRO S1 Units/1(max_flow_per_unit)
  PRO S1 Feed Minimum_gpm/1 -> Switch/3
  Actual S1 Concentrate_gpm/1 -> Actual S2 Concentrate_gpm/1
  UF Flow Maximum_gpm/1 -> Number UF Units/1(max_flow_per_unit)
  Number UF Units/2(Number_in_service) -> [UF_UnitsinService_Request]
  Number PRO S1 Units/2(Number_in_service) -> Scope/1, [PRO_UnitsinService_Request]
  Controls/8 -> [T]  "Temperature (oC)"
  Controls/7 -> uS > mg/L/2  "S1 Feed Conductivity (uS/cm)"
  [sal] -> uS > mg/L/1
  uS > mg/L/1 -> mg/L>g/L/1  "Feed Conductivity (mg/L)"
  mg/L>g/L/1 -> [PROS1_FeedTDS_gL]  "S1 Feed Salinity (g/L)"
  Number UF Units/1(flows) -> UF_UnitDispatch/1, [UF_FlowsperUnit_Vector], Delay One Step/1
  Number PRO S1 Units/1(flows) -> [PRO_FlowperUnit_gpm], PRO_UnitDispatch/1, Display/1, Unit Delay/1
  Constant7/1 -> Gain2/1
  Constant/1 -> Minus/1
  Minus/1 -> TSRO Feed Setpoint/2, Actual S2 Concentrate_gpm/2
  Constant1/1 -> Minus1/1
  Minus1/1 -> Product/2, Actual S1 Concentrate_gpm/2
  SolarImport/1 -> Solar Scenario/1
  Constant8/1 -> Gain3/1
  TOURateImport/2 -> [TOURates], Scope2/1
  Controls/1 -> Switch/1, Compare To Constant/1, Scope2/2, Bus Creator1/1, UFFiltrateFlow_gpm/2, Saturation2/1, Plant_SetpointvsActual/1  "Plant Feed Setpoint"
  Compare To Constant/1 -> Integrator/2
  Constant2/1 -> Integrator/1
  Integrator/1 -> [Plant_StabilizationTime], Number PRO S1 Units/5(Stabilization_Time), Scope3/1, Switch/2  "Stabilization Time"
  Step/1 -> Integrator/3
  Switch/1 -> Rate Limiter/1  "Plant Feed, Actual"
  Rate Limiter/1 -> Plant_SetpointvsActual/2, Bus Creator1/2, Actual PRO Feed_gpm/1, Saturation1/1  "Plant Feed Actual"
  Solar Scenario/1 -> Max/1
  Max/1 -> Scope2/3, [Plant_SolarPower_kW]
  Constant3/1 -> Max/2
  Unit Delay/1 -> Number PRO S1 Units/4(prev_flows)
  UFFiltrateFlow_gpm/1 -> Product/1, Number PRO S1 Units/3(flow_setpoint)  "ROFeed Setpoint"
  Constant4/1 -> Number PRO S1 Units/6(ROstabilization_time)
  Product/1 -> TSRO Feed Setpoint/1
  TSRO Feed Setpoint/1 -> [TSRO_Flow_SP]
  Delay One Step/1 -> Number UF Units/4(prev_flows)
  Bus Creator1/1 -> [UF_FeedFlow]
  Saturation1/1 -> Number UF Units/2(flow_actual)
  Saturation2/1 -> Number UF Units/3(flow_setpoint)
  Constant6/1 -> Gain1/1
  Gain/1 -> Minus1/2, [PROS1_RR]
  Gain1/1 -> UFFiltrateFlow_gpm/1
  Gain2/1 -> Minus/2, [PROS2_RR]
  Gain3/1 -> [TSRO_RR]
  Controls/9 -> [FeedTurbidity_NTU]  "Temperature (oC)"
